simulink model "Recv4sFlow"  (R2018b)
settings: Solver=FixedStepDiscrete  StartTime=0.0  StopTime=10.0  FixedStep=0.01  RelTol=1e-3
settings Model: Creator=sn2xws  LastModifiedBy=sn2xws
settings DataIOCC: SaveFormat=StructureWithTime
settings OptimizationCC: DefaultParameterBehavior=Inlined  EnhancedBackFolding=on  PassReuseOutputArgsAs=Individual arguments  ZeroExternalMemoryAtStartup=off  ZeroInternalMemoryAtStartup=off  OptimizeBlockOrder=speed  DifferentSizesBufferReuse=on  OptimizationCustomize=off
settings DebuggingCC: ParameterTunabilityLossMsg=error
settings SFSimCC: MATLABDynamicMemAlloc=off
settings RTWCC: SystemTargetFile=autosar.tlc  GenCodeOnly=on  TemplateMakefile=ert_default_tmf  Description=AUTOSAR  GenerateReport=on  IncludeHyperlinkInReport=on  LaunchReport=on  GenerateTraceInfo=on  GenerateTraceReport=on  GenerateTraceReportSl=on  GenerateTraceReportSf=on  GenerateTraceReportEml=on  GenerateCodeMetricsReport=on
settings CodeAppCC: ForceParamTrailComments=on  IgnoreCustomStorageClasses=off  OperatorAnnotations=on  SimulinkDataObjDesc=on  SFDataObjDesc=on  InsertBlockDesc=on
settings STFCustomTargetCC: TargetLangStandard=C99 (ISO)  MultiwordLength=256  ParMdlRefBuildCompliant=on  CompOptLevelCompliant=on  IncludeMdlTerminateFcn=off  CombineOutputUpdateFcns=on  SuppressErrorStatus=on  ERTCustomFileBanners=on  SupportNonFinite=off  SupportComplex=off  SupportContinuousTime=off  SupportNonInlinedSFcns=off  RemoveResetFunc=on  MATLABClassNameForMDSCustomization=Simulink.SoftwareTarget.ERTCustomization  AutosarCompliant=on  UseToolchainInfoCompliant=on  LookupTableObjectStructAxisOrder=2,1,3,4,...  LUTObjectStructOrderEvenSpacing=Size,Table,Breakpoints  SystemTargetFile=autosar.tlc
settings ERTTargetCC: TargetLangStandard=C99 (ISO)  ConcurrentExecutionCompliant=off  IncludeMdlTerminateFcn=off  SuppressErrorStatus=on  SupportNonFinite=off  SupportComplex=off  ModelStepFunctionPrototypeControlCompliant=off  CPPClassGenCompliant=off  AutosarCompliant=on  LookupTableObjectStructAxisOrder=2,1,3,4,...  LUTObjectStructOrderEvenSpacing=Size,Table,Breakpoints  InlinedParameterPlacement=NonHierarchical  ERTCustomFileTemplate=example_file_process.tlc  ERTFilePackagingFormat=Compact

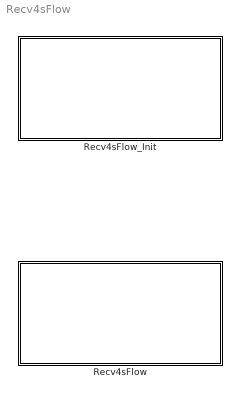
== system Recv4sFlow ==
  Recv4sFlow : Subsystem
  Recv4sFlow_Init : Subsystem

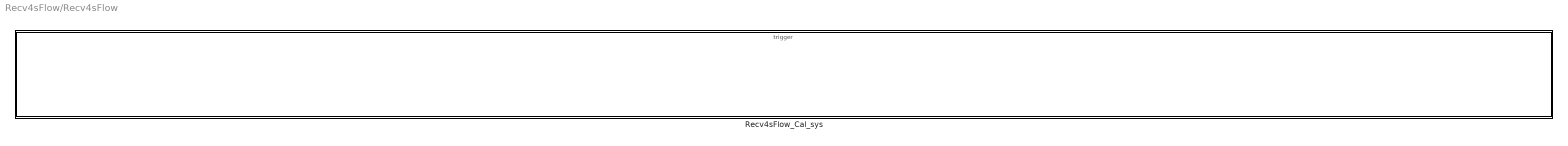
== system Recv4sFlow/Recv4sFlow ==
  Recv4sFlow_Cal_sys : Subsystem

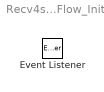
== system Recv4sFlow/Recv4sFlow_Init ==
  Event Listener : EventListener  EventName=reset

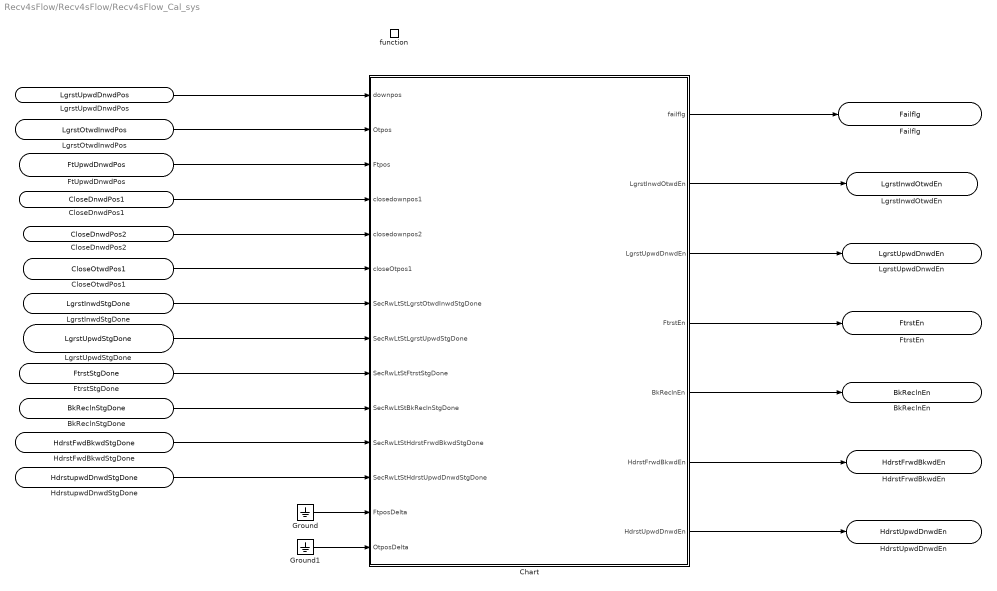
== system Recv4sFlow/Recv4sFlow/Recv4sFlow_Cal_sys ==
  function : TriggerPort  TriggerType=function-call  IsSimulinkFunction=on  FunctionName=Recv4sFlow_Cal  VariantControl=(inherit)
  Chart : Stateflow chart  TreatAsAtomicUnit=on
  Ground : Ground
  Ground1 : Ground
  LgrstUpwdDnwdPos : ArgIn  OutDataTypeStr=uint16  ArgumentName=LgrstUpwdDnwdPos
  LgrstOtwdInwdPos : ArgIn  Port=2  OutDataTypeStr=uint16  ArgumentName=LgrstOtwdInwdPos
  FtUpwdDnwdPos : ArgIn  Port=3  OutDataTypeStr=uint16  ArgumentName=FtUpwdDnwdPos
  CloseDnwdPos1 : ArgIn  Port=4  OutDataTypeStr=uint16  ArgumentName=CloseDnwdPos1
  CloseDnwdPos2 : ArgIn  Port=5  OutDataTypeStr=uint16  ArgumentName=CloseDnwdPos2
  CloseOtwdPos1 : ArgIn  Port=6  OutDataTypeStr=uint16  ArgumentName=CloseOtwdPos1
  LgrstInwdStgDone : ArgIn  Port=7  OutDataTypeStr=boolean  ArgumentName=LgrstInwdStgDone
  LgrstUpwdStgDone : ArgIn  Port=8  OutDataTypeStr=boolean  ArgumentName=LgrstUpwdStgDone
  FtrstStgDone : ArgIn  Port=9  OutDataTypeStr=boolean  ArgumentName=FtrstStgDone
  BkReclnStgDone : ArgIn  Port=10  OutDataTypeStr=boolean  ArgumentName=BkReclnStgDone
  HdrstFwdBkwdStgDone : ArgIn  Port=11  OutDataTypeStr=boolean  ArgumentName=HdrstFwdBkwdStgDone
  HdrstupwdDnwdStgDone : ArgIn  Port=12  OutDataTypeStr=boolean  ArgumentName=HdrstupwdDnwdStgDone
  Failflg : ArgOut  OutDataTypeStr=boolean  ArgumentName=Failflg
  LgrstInwdOtwdEn : ArgOut  Port=2  OutDataTypeStr=boolean  ArgumentName=LgrstInwdOtwdEn
  LgrstUpwdDnwdEn : ArgOut  Port=3  OutDataTypeStr=boolean  ArgumentName=LgrstUpwdDnwdEn
  FtrstEn : ArgOut  Port=4  OutDataTypeStr=boolean  ArgumentName=FtrstEn
  BkReclnEn : ArgOut  Port=5  OutDataTypeStr=boolean  ArgumentName=BkReclnEn
  HdrstFrwdBkwdEn : ArgOut  Port=6  OutDataTypeStr=boolean  ArgumentName=HdrstFrwdBkwdEn
  HdrstUpwdDnwdEn : ArgOut  Port=7  OutDataTypeStr=boolean  ArgumentName=HdrstUpwdDnwdEn
  wires:
  CloseDnwdPos2/1 -> Chart/5(closedownpos2)
  BkReclnStgDone/1 -> Chart/10(SecRwLtStBkReclnStgDone)
  HdrstFwdBkwdStgDone/1 -> Chart/11(SecRwLtStHdrstFrwdBkwdStgDone)
  HdrstupwdDnwdStgDone/1 -> Chart/12(SecRwLtStHdrstUpwdDnwdStgDone)
  LgrstUpwdDnwdPos/1 -> Chart/1(downpos)
  CloseDnwdPos1/1 -> Chart/4(closedownpos1)
  CloseOtwdPos1/1 -> Chart/6(closeOtpos1)
  LgrstInwdStgDone/1 -> Chart/7(SecRwLtStLgrstOtwdInwdStgDone)
  FtrstStgDone/1 -> Chart/9(SecRwLtStFtrstStgDone)
  LgrstOtwdInwdPos/1 -> Chart/2(Otpos)
  FtUpwdDnwdPos/1 -> Chart/3(Ftpos)
  LgrstUpwdStgDone/1 -> Chart/8(SecRwLtStLgrstUpwdStgDone)
  Chart/1(failflg) -> Failflg/1
  Chart/2(LgrstInwdOtwdEn) -> LgrstInwdOtwdEn/1
  Chart/3(LgrstUpwdDnwdEn) -> LgrstUpwdDnwdEn/1
  Chart/4(FtrstEn) -> FtrstEn/1
  Chart/5(BkReclnEn) -> BkReclnEn/1
  Chart/6(HdrstFrwdBkwdEn) -> HdrstFrwdBkwdEn/1
  Chart/7(HdrstUpwdDnwdEn) -> HdrstUpwdDnwdEn/1
  Ground/1 -> Chart/13(FtposDelta)
  Ground1/1 -> Chart/14(OtposDelta)

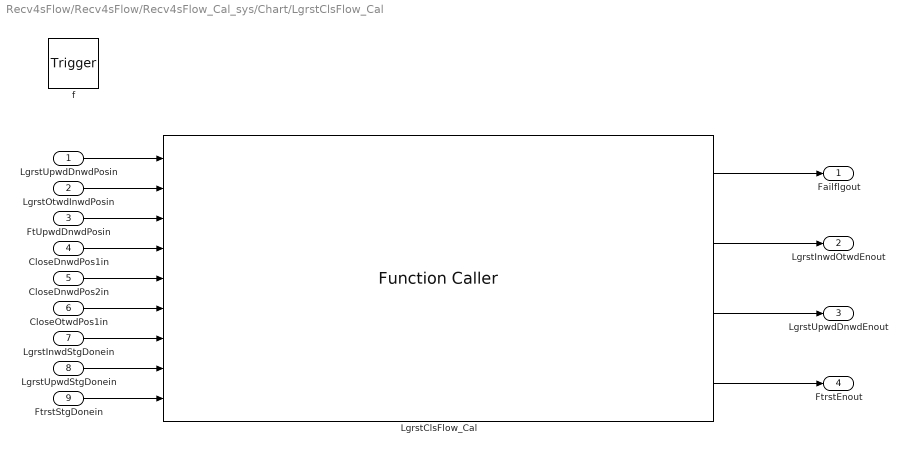
== system Recv4sFlow/Recv4sFlow/Recv4sFlow_Cal_sys/Chart/LgrstClsFlow_Cal ==
  LgrstUpwdDnwdPosin : Inport
  LgrstOtwdInwdPosin : Inport  Port=2
  FtUpwdDnwdPosin : Inport  Port=3
  CloseDnwdPos1in : Inport  Port=4
  CloseDnwdPos2in : Inport  Port=5
  CloseOtwdPos1in : Inport  Port=6
  LgrstInwdStgDonein : Inport  Port=7
  LgrstUpwdStgDonein : Inport  Port=8
  FtrstStgDonein : Inport  Port=9
  f : TriggerPort  TriggerType=function-call  VariantControl=(inherit)
      settings: CopyFcn=Stateflow.SLINSF.SimulinkMan.removeBlockPreDeleteFcn  PreDeleteFcn=Stateflow.SLINSF.SimulinkMan.unsafePredeleteFcn
  LgrstClsFlow_Cal : FunctionCaller  FunctionPrototype=[Failflg,LgrstInwdOtwdEn,LgrstUpwdDnwdEn,FtrstEn] = LgrstClsFlow_Cal(LgrstUpwdDnwdPos,LgrstOtwdInwdPos,FtUpwdDnwdPos,CloseDnwdPos1,CloseDnwdPos2,CloseOtwdPos1,LgrstInwdStgDone,LgrstUpwdStgDone,FtrstStgDone)  InputArgumentSpecifications=uint16(1), uint16(1), uint16(1), uint16(1), uint16(1), uint16(1), boolean(true), boolean(true), boolean(true)  OutputArgumentSpecifications=boolean(true), boolean(true), boolean(true), boolean(true)
  Failflgout : Outport
  LgrstInwdOtwdEnout : Outport  Port=2
  LgrstUpwdDnwdEnout : Outport  Port=3
  FtrstEnout : Outport  Port=4
  wires:
  LgrstUpwdDnwdPosin/1 -> LgrstClsFlow_Cal/1
  LgrstOtwdInwdPosin/1 -> LgrstClsFlow_Cal/2
  FtUpwdDnwdPosin/1 -> LgrstClsFlow_Cal/3
  CloseDnwdPos1in/1 -> LgrstClsFlow_Cal/4
  CloseDnwdPos2in/1 -> LgrstClsFlow_Cal/5
  CloseOtwdPos1in/1 -> LgrstClsFlow_Cal/6
  LgrstInwdStgDonein/1 -> LgrstClsFlow_Cal/7
  LgrstUpwdStgDonein/1 -> LgrstClsFlow_Cal/8
  FtrstStgDonein/1 -> LgrstClsFlow_Cal/9
  LgrstClsFlow_Cal/1 -> Failflgout/1
  LgrstClsFlow_Cal/2 -> LgrstInwdOtwdEnout/1
  LgrstClsFlow_Cal/3 -> LgrstUpwdDnwdEnout/1
  LgrstClsFlow_Cal/4 -> FtrstEnout/1

== stateflow chart Recv4sFlow/Recv4sFlow_Cal_sys/Chart ==
  state [Failflgout,LgrstInwdOtwdEnout,LgrstUpwdDnwdEnout,FtrstEnout] = LgrstClsFlow_Cal(LgrstUpwdDnwdPosin,LgrstOtwdInwdPosin,FtUpwdDnwdPosin,CloseDnwdPos1in,CloseDnwdPos2in,CloseOtwdPos1in,LgrstInwdStgDonein,LgrstUpwdStgDonein,FtrstStgDonein) [function]
  (default) -> (junction 5) : {
      | failflg=0;
      | LgrstInwdOtwdEn = 0;
      | LgrstUpwdDnwdEn=0;
      | FtrstEn = 0;
      | BkReclnEn = 0;
      | HdrstFrwdBkwdEn = 0;
      | HdrstUpwdDnwdEn = 0;
      | }
  (junction 5) -> (junction 9) [order 1] : [SecRwLtStBkReclnStgDone]
  (junction 5) -> (junction 7) [order 2] : {BkReclnEn=1;}
  (junction 9) -> (junction 11)
  (junction 11) -> (junction 7)
  (junction 7) -> (junction 244)
  (junction 244) -> (junction 234) [order 1] : [SecRwLtStHdrstUpwdDnwdStgDone]
  (junction 244) -> (junction 246) [order 2] : {HdrstUpwdDnwdEn=1;}
  (junction 234) -> (junction 236)
  (junction 236) -> (junction 246)
  (junction 246) -> (junction 182) : {[failflg,LgrstInwdOtwdEn,LgrstUpwdDnwdEn,FtrstEn] = LgrstClsFlow_Cal(downpos,Otpos,Ftpos,closedownpos1,closedownpos2,closeOtpos1,SecRwLtStLgrstOtwdInwdStgDone,SecRwLtStLgrstUpwdStgDone,SecRwLtStFtrstStgDone);}
  (junction 182) -> (junction 252) [order 1] : [(SecRwLtStLgrstOtwdInwdStgDone&&SecRwLtStLgrstUpwdStgDone&&SecRwLtStFtrstStgDone)||failflg==1]
  (junction 252) -> (junction 173) [order 1] : [SecRwLtStHdrstFrwdBkwdStgDone]
  (junction 182) -> (junction 181) [order 2]
  (junction 252) -> (junction 254) [order 2] : {HdrstFrwdBkwdEn = 1;}
  (junction 173) -> (junction 175)
  (junction 254) -> (junction 181)
  (junction 175) -> (junction 254)
  (junction 181) -> (junction 165)
  data: LgrstUpwdDnwdPosin function_input; LgrstOtwdInwdPosin function_input; FtUpwdDnwdPosin function_input; CloseDnwdPos1in function_input; CloseDnwdPos2in function_input; CloseOtwdPos1in function_input; LgrstInwdStgDonein function_input; LgrstUpwdStgDonein function_input; FtrstStgDonein function_input; Failflgout function_output; LgrstInwdOtwdEnout function_output; LgrstUpwdDnwdEnout function_output; FtrstEnout function_output; downpos input uint16; Otpos input uint16; Ftpos input uint16; closedownpos1 input uint16; closedownpos2 input uint16; closeOtpos1 input uint16; SecRwLtStLgrstOtwdInwdStgDone input boolean; SecRwLtStLgrstUpwdStgDone input boolean; SecRwLtStFtrstStgDone input boolean; SecRwLtStBkReclnStgDone input boolean; SecRwLtStHdrstFrwdBkwdStgDone input boolean; SecRwLtStHdrstUpwdDnwdStgDone input boolean; FtposDelta input uint16; OtposDelta input uint16; failflg output boolean; LgrstInwdOtwdEn output boolean; LgrstUpwdDnwdEn output boolean; FtrstEn output boolean; BkReclnEn output boolean; HdrstFrwdBkwdEn output boolean; HdrstUpwdDnwdEn output boolean
